simulink model "ElectricalThermalSystemSSC"  (R2026b)
settings: Solver=VariableStepAuto
undefined symbols (not defined in the file): coolant_pipe_D, coolant_valve_D_ratio_max, coolant_valve_D_ratio_min, coolant_valve_displacement, EnvAirTemp, EnvGrvty, PlntThrCabCO2Init, PlntThrCabDucArea, PlntThrCabFanMaxFlw, PlntThrCabHtc, PlntThrCabNPass, PlntThrCabRelHInit, PlntThrCabTempAvg, PlntThrChArea, PlntThrCmpMaxSpd, PlntThrCoolTnkArea, PlntThrCoolTnkVol, PlntThrDoorsArea, PlntThrDoorsK, PlntThrDoorsTk, PlntThrExpDia, PlntThrFanMaxSpd, PlntThrFanMechEff, PlntThrFanVolEff, PlntThrGlassArea, PlntThrGlassK, PlntThrGlassTk, PlntThrHeaterMaxPwr, PlntThrHexNTubes, PlntThrHexTubeDia, PlntThrPipeArea, PlntThrPipeDia, PlntThrPmpMaxSpd, PlntThrPTCLimTemp, PlntThrPTCPwrGain, PlntThrRefrigDia, PlntThrRefrigPinit, PlntThrRoofArea, PlntThrRoofK, PlntThrRoofTk, PlntThrValDisp, PlntThrValDratioMax, PlntThrValDratioMin, PlntThrValRefrDisp, PlntThrValRefrDratio, PlntThrValSplMax, ThrmEM1, ThrmEM2, ThrmEM3, ThrmEM4
libraries: fl_lib x149, nesl_utility x81, SimscapeFluids_lib x35, autolibutils x21
(part 4 of 6)

== system ElectricalThermalSystemSSC/Heater ==
  1 : Inport
  Battery Heater : fl_lib/Thermal/Thermal Elements/Thermal Mass  mass_type=foundation.enum.constant_variable.constant  mass=2 kg  sp_heat=447 J/kg/K  mass_min=1e-6 kg  num_ports=foundation.enum.numPorts2.one  m_specify=off  m_priority=High  m=1 kg  m_nominal_specify=off  m_nominal_value=1  m_nominal_unit=kg  T_specify=on  T_priority=High  T=EnvAirTemp K  T_nominal_specify=off  T_nominal_value=1  T_nominal_unit=K  Q_specify=off  Q_priority=None  Q=0 W  Q_nominal_specify=off  Q_nominal_value=1  Q_nominal_unit=W
  Controlled Heat Flow Rate Source : fl_lib/Thermal/Thermal Sources/Controlled Heat Flow Rate Source
  Convective Heat Transfer : fl_lib/Thermal/Thermal Elements/Convective Heat Transfer  thermal_type=foundation.enum.constant_variable.constant  area=PlntThrHeaterJacArea m^2  heat_tr_coeff=PlntThrHeaterCoeff W/(m^2 * K)  min_heat_tr_coeff=1e-3 W/(K*m^2)  T_specify=off  T_priority=None  T=0 K  T_nominal_specify=off  T_nominal_value=1  T_nominal_unit=K  Q_specify=off  Q_priority=None  Q=0 W  Q_nominal_specify=off  Q_nominal_value=1  Q_nominal_unit=W
  Flow Resistance (TL) : fl_lib/Thermal Liquid/Elements/Flow Resistance (TL)  delta_p_nominal=2e-4 MPa  mdot_nominal=0.15 kg/s  area=PlntThrPipeArea m^2  laminar_fraction=1e-3
  Flow Resistance (TL)1 : fl_lib/Thermal Liquid/Elements/Flow Resistance (TL)  delta_p_nominal=2e-4 MPa  mdot_nominal=0.15 kg/s  area=PlntThrPipeArea m^2  laminar_fraction=1e-3
  Heater Coolant Volume : fl_lib/Thermal Liquid/Elements/Constant Volume Chamber (TL)  volume=PlntThrHeaterJacVol m^3  num_ports=foundation.enum.num_ports.two  area_A=PlntThrPipeArea m^2  area_B=PlntThrPipeArea m^2  area_C=0.01 m^2  area_D=0.01 m^2  p_I_specify=on  p_I_priority=High  p_I=EnvAbsPrs Pa  p_I_nominal_specify=off  p_I_nominal_value=1  p_I_nominal_unit=MPa  T_I_specify=on  T_I_priority=High  T_I=EnvAirTemp K  T_I_nominal_specify=off  T_I_nominal_value=1  T_I_nominal_unit=K  u_I_specify=off  u_I_priority=None  u_I=83.90600000000001 kJ/kg  u_I_nominal_specify=off  u_I_nominal_value=1  u_I_nominal_unit=kJ/kg  rho_I_specify=off  rho_I_priority=None  rho_I=998.21 kg/m^3  rho_I_nominal_specify=off  rho_I_nominal_value=1  rho_I_nominal_unit=kg/m^3
  LPF with IC1 : Subsystem  mask{wc=1, InitCond=0, dataType=off}
      mask prompts: wc "Cutoff frequency, wc [rad/s]"; InitCond "Initial condition, InitCond [same as u]"; dataType "Enforce same input data type"
      mask TypeOptions wc: Cont LPF IC/wc
      mask TypeOptions InitCond: Initial Condition/Value
      mask TypeOptions dataType: Cont LPF IC/dataType
  Max Power [W] : Gain  Gain=PlntThrHeaterMaxPwr
  Signal Specification : SignalSpecification  Unit=W
  Simulink-PS Converter : nesl_utility/Simulink-PS Converter  PhysicalDomain=network_engine_domain  SubClassName=ps_input  LeftPortType=input  RightPortType=output  PseudoPeriodic=off  Frequencies=[]  NoiseDistribution=none  NoiseParameters=[]  Unit=W  AffineConversion=off  FilteringAndDerivatives=provide  SimscapeFilterOrder=1  InputFilterTimeConstant=0.001  UdotUserProvided=0
  Thermal Reference : fl_lib/Thermal/Thermal Elements/Thermal Reference
  B : PMIOPort  Side=Left
  A : PMIOPort  Port=2  Side=Right
  01 : Outport
  wires:
  1/1 -> LPF with IC1/1(u)
  LPF with IC1/1(y) -> Max Power [W]/1
  Max Power [W]/1 -> Signal Specification/1, Simulink-PS Converter/1
  Signal Specification/1 -> 01/1
  connections:
  Battery Heater/LConn1 -- Controlled Heat Flow Rate Source/LConn1 -- Convective Heat Transfer/LConn1
  Convective Heat Transfer/RConn1 -- Heater Coolant Volume/LConn2
  Simulink-PS Converter/RConn1 -- Controlled Heat Flow Rate Source/RConn1
  Flow Resistance (TL)/LConn1 -- A/RConn1
  Flow Resistance (TL)1/RConn1 -- B/RConn1
  Flow Resistance (TL)1/LConn1 -- Heater Coolant Volume/RConn1
  Flow Resistance (TL)/RConn1 -- Heater Coolant Volume/LConn1
  Thermal Reference/LConn1 -- Controlled Heat Flow Rate Source/RConn2

== system ElectricalThermalSystemSSC/Inner Condenser ==
  Inner Condenser : SimscapeFluids_lib/Heat Exchangers/Two-Phase Fluid - Moist Air/Condenser Evaporator (2P-MA)  flow_arrangement=fluids.heat_exchangers.enum.FlowArrangement2PMA.Cross  cross_flow_arrangement=fluids.heat_exchangers.enum.CrossFlowArrangement2PMA.UnmixedUnmixed  R_wall=PlntThrICondThermalR K/kW  wall_thermal_mass=false  mass_wall=1 kg  cp_wall=490 J/(K*kg)  area_A1=PlntThrRefrigArea m^2  area_B1=PlntThrRefrigArea m^2  area_A2=PlntThrCabDucArea m^2  area_B2=PlntThrCabDucArea m^2  tube_num_2P=PlntThrICondNTubes  tube_length_2P=PlntThrICondLen m  tube_cross_section_2P=fluids.heat_exchangers.enum.TubeCrossSection.Rectangular  tube_diameter_2P=0.05 m  tube_width_2P=PlntThrICondWdt m  tube_height_2P=PlntThrICondTubHgt m  tube_inner_diameter_2P=0.05 m  tube_outer_diameter_2P=0.1 m  tube_flow_area_2P=0.002 m^2  tube_wetted_perimeter_2P=0.15 m  tube_heat_perimeter_2P=0.15 m  tube_pressure_loss_spec_2P=fluids.heat_exchangers.enum.TubePressureLossSpec2P.Haaland  tube_loss_coeff_2P=10  tube_local_pressure_loss_spec_2P=fluids.heat_exchangers.enum.LocalLossSpec.AggregateLength  tube_length_add_2P=PlntThrICondTubLEq m  tube_local_loss_coefficient_2P=0.1  tube_roughness_pressure_2P=15e-6 m  tube_Re_lam_pressure_2P=2000  tube_Re_tur_pressure_2P=4000  tube_shape_factor_generic_2P=64  tube_heat_coeff_spec_2P=fluids.heat_exchangers.enum.TubeHeatCoeffSpec2P.GneilinskiCavalliniZecchin  tube_colburn_coeff_liq_2P=[.023, .8, .33]  tube_colburn_coeff_mix_2P=[.05, .8, .33]  tube_colburn_coeff_vap_2P=[.023, .8, .33]  tube_roughness_heat_2P=15e-6 m  tube_Re_lam_heat_2P=2000  tube_Re_tur_heat_2P=4000  tube_Nu_lam_generic_2P=3.66  fouling_factor_2P=0.1 K*m^2/kW  fin_area_2P=PlntThrICondTubAWb m^2  fin_efficiency_2P=0.6  energy_spec_2P=foundation.enum.energy_spec.void_fraction  p_init_2P=PlntThrRefrigPinit Pa  T_init_2P=293.15 K  x_init_2P=0.5  alpha_init_2P=PlntThrRefrigAinit  h_init_2P=1500 kJ/kg  u_init_2P=1500 kJ/kg  flow_geometry_MA=fluids.heat_exchangers.enum.FlowGeometryMA.Generic  tube_num_MA=25  tube_length_MA=1 m  tube_cross_section_MA=fluids.heat_exchangers.enum.TubeCrossSection.Circular  tube_diameter_MA=0.05 m  tube_width_MA=0.05 m  tube_height_MA=0.05 m  tube_inner_diameter_MA=0.05 m  tube_outer_diameter_MA=0.1 m  tube_flow_area_MA=0.002 m^2  tube_wetted_perimeter_MA=0.15 m  tube_heat_perimeter_MA=0.15 m  tube_pressure_loss_spec_MA=fluids.heat_exchangers.enum.TubePressureLossSpec.Haaland  tube_loss_coeff_MA=10  tube_local_pressure_loss_spec_MA=fluids.heat_exchangers.enum.LocalLossSpec.AggregateLength  tube_length_add_MA=0.1 m  tube_local_loss_coefficient_MA=0.1  tube_roughness_pressure_MA=15e-6 m  tube_Re_lam_pressure_MA=2000  tube_Re_tur_pressure_MA=4000  tube_shape_factor_generic_MA=64  tube_heat_coeff_spec_MA=fluids.heat_exchangers.enum.TubeHeatCoeffSpec.Gneilinski  tube_colburn_coeff_MA=[.023, .8, .33]  tube_roughness_heat_MA=15e-6 m  tube_Re_lam_heat_MA=2000  tube_Re_tur_heat_MA=4000  tube_Nu_lam_generic_MA=3.66  bank_arrangement_MA=fluids.heat_exchangers.enum.BankArrangement.Inline  bank_num_rows_MA=5  bank_tubes_per_row_MA=5  bank_width_MA=1 m  bank_tube_diameter_MA=0.05 m  bank_longitudinal_pitch_MA=0.15 m  bank_transverse_pitch_MA=0.15 m  bank_pressure_loss_spec_MA=fluids.heat_exchangers.enum.BankPressureLossSpec.Martin  bank_euler_MA=10  bank_heat_coeff_spec_MA=fluids.heat_exchangers.enum.BankHeatCoeffSpec.Martin  bank_colburn_coeff_MA=[.27, .63, .36]  generic_flow_area_MA=PlntThrICondAreaFlw m^2  generic_heat_area_MA=PlntThrICondAreaPr m^2  generic_volume_MA=PlntThrICondAirVol m^3  generic_loss_coeff_MA=10  generic_colburn_coeff_MA=[.023, .8, .33]  fouling_factor_MA=0.1 K*m^2/kW  fin_area_MA=PlntThrICondAreaFins m^2  fin_efficiency_MA=0.7  p_init_MA=EnvAbsPrs Pa  T_init_MA=EnvAirTemp K  humidity_spec_MA=foundation.enum.HumiditySpec.RelativeHumidity  RH_init_MA=PlntThrCabRelHInit  x_w_init_MA=0.01  y_w_init_MA=0.01  HR_init_MA=0.01  Tw_init_MA=287 K  trace_gas_spec_MA=foundation.enum.trace_gas_spec.mole_fraction  x_g_init_MA=0.001  y_g_init_MA=PlntThrCabCO2Init  r_d_init_MA=0  RH_ws_MA=1  time_constant_cond_MA=1e-3 s  time_constant_evap_MA=1e-3 s  fraction_entrained_MA=1
  PS-Simulink Converter1 : nesl_utility/PS-Simulink Converter  PhysicalDomain=network_engine_domain  SubClassName=ps_output  LeftPortType=input  RightPortType=output  PseudoPeriodic=off  Frequencies=[]  VectorFormat=inherit  Unit=MPa  AffineConversion=off
  "Pressure, Temperature & Internal Energy Sensor (2P)" : fl_lib/Two-Phase Fluid/Sensors/Pressure, Temperature & Internal Energy Sensor (2P)  reference=foundation.enum.MeasurementReference.absolute  pressure=true  pressure_spec=foundation.enum.PressureMeasementSpec.Absolute  temperature=false  internal_energy=false
  C : PMIOPort  Side=Left
  B : PMIOPort  Port=2  Side=Left
  D : PMIOPort  Port=3  Side=Right
  A : PMIOPort  Port=4  Side=Right
  01 : Outport
  wires:
  PS-Simulink Converter1/1 -> 01/1
  connections:
  PS-Simulink Converter1/LConn1 -- "Pressure, Temperature & Internal Energy Sensor (2P)"/RConn1
  Inner Condenser/LConn3 -- B/RConn1 -- "Pressure, Temperature & Internal Energy Sensor (2P)"/LConn1
  A/RConn1 -- Inner Condenser/LConn1
  C/RConn1 -- Inner Condenser/RConn3
  D/RConn1 -- Inner Condenser/RConn1

== system ElectricalThermalSystemSSC/LPF with IC1 ==
  u : Inport
  Cont LPF IC : autolibutils/Cont LPF IC  wc=wc  aMode=1  dataType=off
  Initial Condition : Constant  Value=InitCond  SampleTime=-1
  y : Outport
  wires:
  Initial Condition/1 -> Cont LPF IC/2
  u/1 -> Cont LPF IC/1
  Cont LPF IC/1 -> y/1

== system ElectricalThermalSystemSSC/Motor ==
  Cooling Assembly : Subsystem  Variant=on  VariantControl=Cooling Assembly  EmptyChoice=on
  PS-Simulink Converter : nesl_utility/PS-Simulink Converter  PhysicalDomain=network_engine_domain  SubClassName=ps_output  LeftPortType=input  RightPortType=output  PseudoPeriodic=off  Frequencies=[]  VectorFormat=inherit  Unit=K  AffineConversion=on
  Pressure & Temperature Sensor (TL) : fl_lib/Thermal Liquid/Sensors/Pressure & Temperature Sensor (TL)  reference=foundation.enum.MeasurementReference.absolute  pressure=false  pressure_spec=foundation.enum.PressureMeasementSpec.Absolute  temperature=true
  Simscape Bus1 : SimscapeBus  HierarchyStrings=ThrmEM4;ThrmEM3;ThrmEM2;ThrmEM1
  A : PMIOPort  Side=Left
  B : PMIOPort  Port=2  Side=Right
  T : PMIOPort  Port=3  Side=Right
  01 : Outport
  02 : Outport  Port=2
  03 : Outport  Port=3
  wires:
  Cooling Assembly/2(Qem) -> 03/1
  PS-Simulink Converter/1 -> 02/1
  Cooling Assembly/1(EMTemp) -> 01/1
  connections:
  Simscape Bus1/LConn1 -- Cooling Assembly/RConn2
  Simscape Bus1/LConn4 -- Cooling Assembly/RConn5
  Simscape Bus1/LConn3 -- Cooling Assembly/RConn4
  Pressure & Temperature Sensor (TL)/LConn1 -- B/RConn1 -- Cooling Assembly/RConn1
  T/RConn1 -- Simscape Bus1/RConn1
  A/RConn1 -- Cooling Assembly/LConn1
  Simscape Bus1/LConn2 -- Cooling Assembly/RConn3
  PS-Simulink Converter/LConn1 -- Pressure & Temperature Sensor (TL)/RConn1

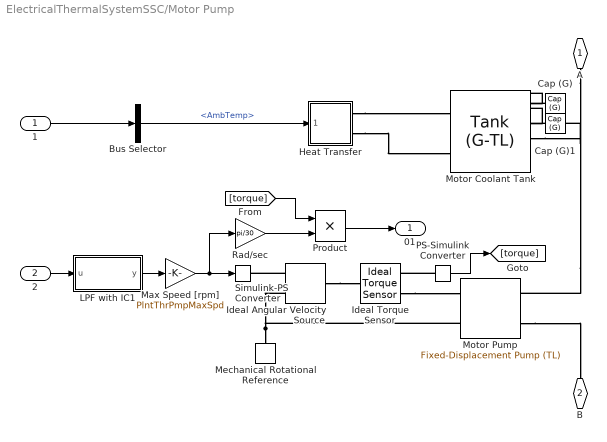
== system ElectricalThermalSystemSSC/Motor Pump ==
  1 : Inport
  2 : Inport  Port=2
  Bus Selector : BusSelector  OutputSignals=AmbTemp
  Cap (G) : fl_lib/Gas/Elements/Cap (G)  p_specify=off  p_priority=None  p=0.101325 MPa  p_nominal_specify=off  p_nominal_value=1  p_nominal_unit=MPa  T_specify=off  T_priority=None  T=293.15 K  T_nominal_specify=off  T_nominal_value=1  T_nominal_unit=K
  Cap (G)1 : fl_lib/Gas/Elements/Cap (G)  p_specify=off  p_priority=None  p=0.101325 MPa  p_nominal_specify=off  p_nominal_value=1  p_nominal_unit=MPa  T_specify=off  T_priority=None  T=293.15 K  T_nominal_specify=off  T_nominal_value=1  T_nominal_unit=K
  Heat Transfer : Subsystem
  Ideal Angular Velocity Source : fl_lib/Mechanical/Mechanical Sources/Ideal Angular Velocity Source
  Ideal Torque Sensor : fl_lib/Mechanical/Mechanical Sensors/Ideal Torque Sensor
  LPF with IC1 : Subsystem  mask{wc=1, InitCond=0, dataType=off}
      mask prompts: wc "Cutoff frequency, wc [rad/s]"; InitCond "Initial condition, InitCond [same as u]"; dataType "Enforce same input data type"
      mask TypeOptions wc: Cont LPF IC/wc
      mask TypeOptions InitCond: Initial Condition/Value
      mask TypeOptions dataType: Cont LPF IC/dataType
  Max Speed [rpm] : Gain  Gain=PlntThrPmpMaxSpd
  Mechanical Rotational Reference : fl_lib/Mechanical/Rotational Elements/Mechanical Rotational Reference
  Motor Coolant Tank : SimscapeFluids_lib/Thermal Liquid/Tanks & Accumulators/Tank (G-TL)  num_inlet=2  volume_total=PlntThrCoolTnkVol l  volume_spec=1  tank_area=PlntThrCoolTnkArea m^2  level_TLU=[0, 3, 5] m  volume_TLU=[0, 4, 6] m^3  inlet_areas_A1B1=[.01, .01] m^2  inlet_height_A2=0.1 m  inlet_area_A2=0.01 m^2  inlet_heights_A2B2=[0, 0] m  inlet_areas_A2B2=[1 1] *PlntThrPipeArea m^2  inlet_heights_A2B2C2=[.1, .05, 0] m  inlet_areas_A2B2C2=[.01, .01, .01] m^2  inlet_heights_A2B2C2D2=0.1 * ones(1, 4) m  inlet_areas_A2B2C2D2=0.01 * ones(1, 4) m^2  inlet_heights_A2B2C2D2E2=0.1 * ones(1, 5) m  inlet_areas_A2B2C2D2E2=0.01 * ones(1, 5) m^2  inlet_heights_A2B2C2D2E2F2=0.1 * ones(1, 6) m  inlet_areas_A2B2C2D2E2F2=0.01 * ones(1, 6) m^2  capacity_check=0  max_liquid_capacity=coolant_tank_volume l  g=0 m/s^2  level_specify=on  level_priority=None  level=5 m  level_nominal_specify=off  level_nominal_value=1  level_nominal_unit=m  volume_liquid_specify=on  volume_liquid_priority=High  volume_liquid=0.5 * PlntThrCoolTnkVol l  volume_liquid_nominal_specify=off  volume_liquid_nominal_value=1  volume_liquid_nominal_unit=m^3  mass_liquid_specify=off  mass_liquid_priority=None  mass_liquid=5e+3 kg  mass_liquid_nominal_specify=off  mass_liquid_nominal_value=1  mass_liquid_nominal_unit=kg  T_liquid_specify=on  T_liquid_priority=High  T_liquid=EnvAirTemp K  T_liquid_nominal_specify=off  T_liquid_nominal_value=1  T_liquid_nominal_unit=K  p_gas_specify=on  p_gas_priority=High  p_gas=EnvAbsPrs Pa  p_gas_nominal_specify=off  p_gas_nominal_value=1  p_gas_nominal_unit=MPa  T_gas_specify=on  T_gas_priority=High  T_gas=EnvAirTemp K  T_gas_nominal_specify=off  T_gas_nominal_value=1  T_gas_nominal_unit=K  rho_gas_specify=off  rho_gas_priority=None  rho_gas=1.2 kg/m^3  rho_gas_nominal_specify=off  rho_gas_nominal_value=1  rho_gas_nominal_unit=kg/m^3
  Motor Pump : SimscapeFluids_lib/Thermal Liquid/Pumps & Motors/Fixed-Displacement Pump (TL)  loss_spec=1  displacement=PlntThrPmpDisp l/rev  omega_nominal=0.5 * PlntThrPmpMaxSpd rpm  p_nominal=0.1 MPa  mu_nominal=0.9 cP  vol_eff_nominal=0.92  mech_eff_nominal=0.88  no_load_torque=0.03 N*m  p_diff_eff_TLU=[.1, 1, 2] MPa  omega_eff_TLU=[25, 50, 100, 200, 300, 400] rad/s  vol_eff_TLU=[.816, .908, .954, .977, .981, .984; .325, .663, .831, .916, .925, .946; .137, .568, .78, .892, .893, .91]  mech_eff_TLU=[.996, .996, .996, .996, .996, .996; .988, .989, .989, .989, .989, .99; .981, .981, .982, .982, .983, .984]  p_diff_loss_TLU=[.1, 1, 2] MPa  omega_loss_TLU=[25, 50, 100, 200, 300, 400] rad/s  vol_loss_TLU=[.023, .023, .023, .023, .0285, .032; .0844, .0842, .0845, .084, .1125, .108; .1079, .108, .11, .108, .1605, .18] * 1e-3 m^3/s  mech_loss_TLU=[.002, .002, .002, .002, .002, .002; .0607, .0556, .0556, .0556, .0556, .0505; .1937, .1937, .1833, .1833, .1729, .1626] N*m  vol_eff_min=1e-3  vol_eff_max=1  mech_eff_min=1e-3  mech_eff_max=1  pressure_threshold=1e-3 MPa  omega_threshold=10 rad/s  area=PlntThrPipeArea m^2  supplied_range_check=0  pump_mode_check=simscape.enum.assert.action.none  pressure_check=simscape.enum.assert.action.none  p_min_valid=0.101325 MPa
  PS-Simulink Converter : nesl_utility/PS-Simulink Converter  PhysicalDomain=network_engine_domain  SubClassName=ps_output  LeftPortType=input  RightPortType=output  PseudoPeriodic=off  Frequencies=[]  VectorFormat=inherit  Unit=N*m  AffineConversion=off
  Product : Product
  Rad/sec : Gain  Gain=pi/30
  Simulink-PS Converter : nesl_utility/Simulink-PS Converter  PhysicalDomain=network_engine_domain  SubClassName=ps_input  LeftPortType=input  RightPortType=output  PseudoPeriodic=off  Frequencies=[]  NoiseDistribution=none  NoiseParameters=[]  Unit=rpm  AffineConversion=off  FilteringAndDerivatives=provide  SimscapeFilterOrder=1  InputFilterTimeConstant=0.001  UdotUserProvided=0
  A : PMIOPort  Side=Left
  B : PMIOPort  Port=2  Side=Right
  01 : Outport
  wires:
  2/1 -> LPF with IC1/1(u)
  Bus Selector/1 -> Heat Transfer/1(1)  "<AmbTemp>"
  1/1 -> Bus Selector/1
  LPF with IC1/1(y) -> Max Speed [rpm]/1
  Max Speed [rpm]/1 -> Rad/sec/1, Simulink-PS Converter/1
  PS-Simulink Converter/1 -> [torque]
  Rad/sec/1 -> Product/2
  [torque] -> Product/1
  Product/1 -> 01/1
  connections:
  Mechanical Rotational Reference/LConn1 -- Ideal Angular Velocity Source/RConn2 -- Motor Pump/RConn2
  Motor Pump/LConn2 -- B/RConn1
  Heat Transfer/RConn2 -- Motor Coolant Tank/RConn2
  Cap (G)/LConn1 -- Motor Coolant Tank/LConn1
  Heat Transfer/RConn1 -- Motor Coolant Tank/RConn1
  Motor Coolant Tank/LConn4 -- Motor Pump/LConn1
  A/RConn1 -- Motor Coolant Tank/LConn3
  Cap (G)1/LConn1 -- Motor Coolant Tank/LConn2
  Ideal Angular Velocity Source/RConn1 -- Simulink-PS Converter/RConn1
  Ideal Torque Sensor/RConn1 -- Motor Pump/RConn1
  Ideal Angular Velocity Source/LConn1 -- Ideal Torque Sensor/LConn1
  PS-Simulink Converter/LConn1 -- Ideal Torque Sensor/RConn2

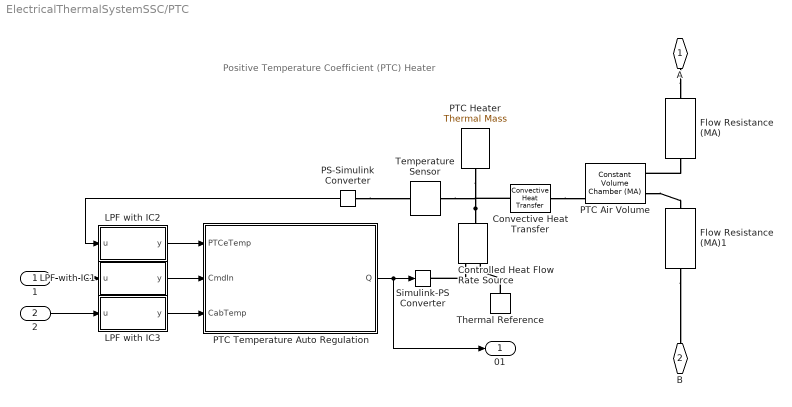
== system ElectricalThermalSystemSSC/PTC ==
  note: Positive Temperature Coefficient (PTC) Heater
  1 : Inport
  2 : Inport  Port=2
  Controlled Heat Flow Rate Source : fl_lib/Thermal/Thermal Sources/Controlled Heat Flow Rate Source
  Convective Heat Transfer : fl_lib/Thermal/Thermal Elements/Convective Heat Transfer  thermal_type=foundation.enum.constant_variable.constant  area=PlntThrPTCArea m^2  heat_tr_coeff=PlntThrPTCHtc W/(m^2 * K)  min_heat_tr_coeff=1e-3 W/(K*m^2)  T_specify=off  T_priority=None  T=0 K  T_nominal_specify=off  T_nominal_value=1  T_nominal_unit=K  Q_specify=off  Q_priority=None  Q=0 W  Q_nominal_specify=off  Q_nominal_value=1  Q_nominal_unit=W
  Flow Resistance (MA) : fl_lib/Moist Air/Elements/Flow Resistance (MA)  delta_p_nominal=2e-4 MPa  mdot_nominal=0.15 kg/s  rho_nominal=1.2 kg/m^3  area=PlntThrCabDucArea m^2  laminar_fraction=1e-3
  Flow Resistance (MA)1 : fl_lib/Moist Air/Elements/Flow Resistance (MA)  delta_p_nominal=2e-4 MPa  mdot_nominal=0.15 kg/s  rho_nominal=1.2 kg/m^3  area=PlntThrCabDucArea m^2  laminar_fraction=1e-3
  LPF with IC1 : Subsystem  mask{wc=1, InitCond=0, dataType=off}
      mask prompts: wc "Cutoff frequency, wc [rad/s]"; InitCond "Initial condition, InitCond [same as u]"; dataType "Enforce same input data type"
      mask TypeOptions wc: Cont LPF IC/wc
      mask TypeOptions InitCond: Initial Condition/Value
      mask TypeOptions dataType: Cont LPF IC/dataType
  LPF with IC2 : Subsystem  mask{wc=10, InitCond=0, dataType=off}
      mask prompts: wc "Cutoff frequency, wc [rad/s]"; InitCond "Initial condition, InitCond [same as u]"; dataType "Enforce same input data type"
      mask TypeOptions wc: Cont LPF IC/wc
      mask TypeOptions InitCond: Initial Condition/Value
      mask TypeOptions dataType: Cont LPF IC/dataType
  LPF with IC3 : Subsystem  mask{wc=1, InitCond=0, dataType=off}
      mask prompts: wc "Cutoff frequency, wc [rad/s]"; InitCond "Initial condition, InitCond [same as u]"; dataType "Enforce same input data type"
      mask TypeOptions wc: Cont LPF IC/wc
      mask TypeOptions InitCond: Initial Condition/Value
      mask TypeOptions dataType: Cont LPF IC/dataType
  PS-Simulink Converter : nesl_utility/PS-Simulink Converter  PhysicalDomain=network_engine_domain  SubClassName=ps_output  LeftPortType=input  RightPortType=output  PseudoPeriodic=off  Frequencies=[]  VectorFormat=inherit  Unit=inherit  AffineConversion=off
  PTC Heater : fl_lib/Thermal/Thermal Elements/Thermal Mass  mass_type=foundation.enum.constant_variable.constant  mass=PlntThrPTCmass kg  sp_heat=PlntThrPTCCp J/kg/K  mass_min=1e-6 kg  num_ports=foundation.enum.numPorts2.one  m_specify=off  m_priority=High  m=1 kg  m_nominal_specify=off  m_nominal_value=1  m_nominal_unit=kg  T_specify=on  T_priority=High  T=EnvAirTemp K  T_nominal_specify=off  T_nominal_value=1  T_nominal_unit=K  Q_specify=off  Q_priority=None  Q=0 W  Q_nominal_specify=off  Q_nominal_value=1  Q_nominal_unit=W
  PTC Air Volume : fl_lib/Moist Air/Elements/Constant Volume Chamber (MA)  volume=0.001 m^3  num_ports=foundation.enum.num_ports.two  area_A=PlntThrCabDucArea m^2  area_B=PlntThrCabDucArea m^2  area_C=0.01 m^2  area_D=0.01 m^2  RH_ws=1  time_constant_cond=1e-3 s  time_constant_evap=1e-3 s  fraction_entrained=1  moisture_trace_gas_source=foundation.enum.moisture_trace_gas_source.none  moisture_source_spec=foundation.enum.MoistureSourceSpec.WaterVapor  vapor_from_liquid=false  moisture_mass_flow=0 kg/s  moisture_temperature_spec=foundation.enum.temperature_spec.atmospheric  moisture_temperature=293.15 K  trace_gas_mass_flow=0 kg/s  trace_gas_temperature_spec=foundation.enum.temperature_spec.atmospheric  trace_gas_temperature=293.15 K  p_init=EnvAbsPrs Pa  p_init_priority=foundation.enum.Priority.High  T_init=EnvAirTemp K  T_init_priority=foundation.enum.Priority.High  humidity_spec=foundation.enum.HumiditySpec.RelativeHumidity  RH_init=PlntThrCabRelHInit  RH_init_priority=foundation.enum.Priority.High  x_w_init=0  x_w_init_priority=foundation.enum.Priority.None  y_w_init=0  y_w_init_priority=foundation.enum.Priority.None  HR_init=0  HR_init_priority=foundation.enum.Priority.None  Tw_init=287 K  Tw_init_priority=foundation.enum.Priority.High  trace_gas_spec=foundation.enum.trace_gas_spec.mole_fraction  x_g_init=0  x_g_init_priority=foundation.enum.Priority.None  y_g_init=PlntThrCabCO2Init  y_g_init_priority=foundation.enum.Priority.High  r_d_init=0  r_d_init_priority=foundation.enum.Priority.High
  PTC Temperature Auto Regulation : Subsystem
  Simulink-PS Converter : nesl_utility/Simulink-PS Converter  PhysicalDomain=network_engine_domain  SubClassName=ps_input  LeftPortType=input  RightPortType=output  PseudoPeriodic=off  Frequencies=[]  NoiseDistribution=none  NoiseParameters=[]  Unit=1  AffineConversion=off  FilteringAndDerivatives=provide  SimscapeFilterOrder=1  InputFilterTimeConstant=0.001  UdotUserProvided=0
  Temperature Sensor : fl_lib/Thermal/Thermal Sensors/Temperature Sensor  temperature_measure=foundation.enum.MeasurementReference.absolute
  Thermal Reference : fl_lib/Thermal/Thermal Elements/Thermal Reference
  A : PMIOPort  Side=Left
  B : PMIOPort  Port=2  Side=Right
  01 : Outport
  wires:
  PTC Temperature Auto Regulation/1(Q) -> 01/1, Simulink-PS Converter/1
  PS-Simulink Converter/1 -> LPF with IC2/1(u)
  1/1 -> LPF with IC1/1(u)
  LPF with IC1/1(y) -> PTC Temperature Auto Regulation/2(CmdIn)
  LPF with IC2/1(y) -> PTC Temperature Auto Regulation/1(PTCeTemp)
  2/1 -> LPF with IC3/1(u)
  LPF with IC3/1(y) -> PTC Temperature Auto Regulation/3(CabTemp)
  connections:
  Controlled Heat Flow Rate Source/RConn1 -- Simulink-PS Converter/RConn1
  PS-Simulink Converter/LConn1 -- Temperature Sensor/RConn1
  A/RConn1 -- Flow Resistance (MA)/LConn1
  PTC Air Volume/LConn2 -- Flow Resistance (MA)1/LConn1
  Flow Resistance (MA)/RConn1 -- PTC Air Volume/LConn1
  Convective Heat Transfer/RConn1 -- PTC Air Volume/RConn3
  Flow Resistance (MA)1/RConn1 -- B/RConn1
  Thermal Reference/LConn1 -- Controlled Heat Flow Rate Source/RConn2
  Controlled Heat Flow Rate Source/LConn1 -- Convective Heat Transfer/LConn1 -- PTC Heater/LConn1 -- Temperature Sensor/LConn1

== system ElectricalThermalSystemSSC/Parallel-Serial Mode Valve 1 ==
  note: Parallel mode flow path: A-C
      | Serial mode flow path: A-B
  1 : Inport
  Bias : Bias  Bias=-1  SaturateOnIntegerOverflow=off
  Gain : Gain  Gain=2
  LPF with IC1 : Subsystem  mask{wc=1, InitCond=0, dataType=off}
      mask prompts: wc "Cutoff frequency, wc [rad/s]"; InitCond "Initial condition, InitCond [same as u]"; dataType "Enforce same input data type"
      mask TypeOptions wc: Cont LPF IC/wc
      mask TypeOptions InitCond: Initial Condition/Value
      mask TypeOptions dataType: Cont LPF IC/dataType
  Max Valve Displacement [m] : Gain  Gain=PlntThrValDisp
  Parallel-Serial Mode Valve : SimscapeFluids_lib/Thermal Liquid/Valves & Orifices/Directional Control Valves/3-Way Directional Valve (TL)  open_orifices_pos=fluids.thermal_liquid.valves.directional_control_valves.enum.OpenOrifices3Way.PA  open_orifices_neg=fluids.thermal_liquid.valves.directional_control_valves.enum.OpenOrifices3Way.AT  area_spec=fluids.thermal_liquid.valves.directional_control_valves.enum.area_spec.identical  valve_spec=fluids.thermal_liquid.valves.enum.orifice_spec.linear  del_S_max=PlntThrValDisp m  area_max=pi * (PlntThrValDratioMax*PlntThrPipeDia)^2 / 4 m^2  del_S_TLU=[0 0.002 0.004 0.007 0.017] m  valve_area_TLU=[1e-09, 2.0352e-07, 4.0736e-05, .00011438, .00034356] m^2  del_S_flow_TLU=[0 0.002 0.004 0.007 0.017] m  p_diff_TLU=[-.1, .3, .5, .7] MPa  vol_flow_TLU=1e-3 * [1.7e-05, 2e-05, 2.6e-05; .0035, .0045, .0053; .7, .9, 1.06; 1.96, 2.5, 3; 6, 7.7, 9.13] m^3/s  mdot_TLU=[-1e-05, 1.7e-05, 2e-05, 2.6e-05; -.002, .0035, .0045, .0053; -.4, .7, .9, 1.06; -1.13, 1.96, 2.5, 3; -3.45, 6, 7.7, 9.13] kg/s  T_ref_in=293.15 K  p_ref_in=0.101325 MPa  area_leak=pi * (PlntThrValDratioMin*PlntThrPipeDia)^2 / 4 m^2  Cd=0.7  Re_c=150  smoothing_factor=0.01  pressure_recovery=simscape.enum.onoff.on  area=PlntThrPipeArea m^2  S_max_PA=PlntThrValSplMax m  del_S_max_PA=coolant_valve_displacement-(coolant_valve_displacement)*(pi * (coolant_valve_D_ratio_min*coolant_pipe_D)^2 / 4)/(pi * (coolant_valve_D_ratio_max*coolant_pipe_D)^2 / 4) m  area_max_PA=pi * (coolant_valve_D_ratio_max*coolant_pipe_D)^2 / 4 m^2  del_S_TLU_PA=[0 0.002 0.004 0.007 0.017] m  valve_area_TLU_PA=[1e-09, 2.0352e-07, 4.0736e-05, .00011438, .00034356] m^2  del_S_flow_TLU_PA=[0 0.002 0.004 0.007 0.017] m  p_diff_TLU_PA=[-.1, .3, .5, .7] MPa  vol_flow_TLU_PA=1e-3 * [1.7e-05, 2e-05, 2.6e-05; .0035, .0045, .0053; .7, .9, 1.06; 1.96, 2.5, 3; 6, 7.7, 9.13] m^3/s  mdot_TLU_PA=[-1e-05, 1.7e-05, 2e-05, 2.6e-05; -.002, .0035, .0045, .0053; -.4, .7, .9, 1.06; -1.13, 1.96, 2.5, 3; -3.45, 6, 7.7, 9.13] kg/s  S_max_AT=-PlntThrValSplMax m  del_S_max_AT=coolant_valve_displacement-(coolant_valve_displacement)*(pi * (coolant_valve_D_ratio_min*coolant_pipe_D)^2 / 4)/(pi * (coolant_valve_D_ratio_max*coolant_pipe_D)^2 / 4) m  area_max_AT=pi * (coolant_valve_D_ratio_max*coolant_pipe_D)^2 / 4 m^2  del_S_TLU_AT=[0 0.002 0.004 0.007 0.017] m  valve_area_TLU_AT=[1e-09, 2.0352e-07, 4.0736e-05, .00011438, .00034356] m^2  del_S_flow_TLU_AT=[0 0.002 0.004 0.007 0.017] m  p_diff_TLU_AT=[-.1, .3, .5, .7] MPa  vol_flow_TLU_AT=1e-3 * [1.7e-05, 2e-05, 2.6e-05; .0035, .0045, .0053; .7, .9, 1.06; 1.96, 2.5, 3; 6, 7.7, 9.13] m^3/s  mdot_TLU_AT=[-1e-05, 1.7e-05, 2e-05, 2.6e-05; -.002, .0035, .0045, .0053; -.4, .7, .9, 1.06; -1.13, 1.96, 2.5, 3; -3.45, 6, 7.7, 9.13] kg/s  S_max_PT=2.5e-3 m  del_S_max_PT=0.005 m  area_max_PT=1e-4 m^2  del_S_TLU_PT=[0, .002, .004, .007, .017] m  valve_area_TLU_PT=[1e-09, 2.0352e-07, 4.0736e-05, .00011438, .00034356] m^2  del_S_flow_TLU_PT=[0, .002, .004, .007, .017] m  p_diff_TLU_PT=[.3, .5, .7] MPa  vol_flow_TLU_PT=1e-3 * [1.7e-05, 2e-05, 2.6e-05; .0035, .0045, .0053; .7, .9, 1.06; 1.96, 2.5, 3; 6, 7.7, 9.13] m^3/s  mdot_TLU_PT=[1.7e-05, 2e-05, 2.6e-05; .0035, .0045, .0053; .7, .9, 1.06; 1.96, 2.5, 3; 6, 7.7, 9.13] kg/s
  Simulink-PS Converter : nesl_utility/Simulink-PS Converter  PhysicalDomain=network_engine_domain  SubClassName=ps_input  LeftPortType=input  RightPortType=output  PseudoPeriodic=off  Frequencies=[]  NoiseDistribution=none  NoiseParameters=[]  Unit=m  AffineConversion=off  FilteringAndDerivatives=provide  SimscapeFilterOrder=1  InputFilterTimeConstant=0.001  UdotUserProvided=0
  C : PMIOPort  Side=Left
  A : PMIOPort  Port=2  Side=Right
  B : PMIOPort  Port=3  Side=Right
  wires:
  1/1 -> LPF with IC1/1(u)
  Gain/1 -> Bias/1
  LPF with IC1/1(y) -> Gain/1
  Max Valve Displacement [m]/1 -> Simulink-PS Converter/1
  Bias/1 -> Max Valve Displacement [m]/1
  connections:
  Parallel-Serial Mode Valve/RConn1 -- Simulink-PS Converter/RConn1
  Parallel-Serial Mode Valve/RConn3 -- C/RConn1
  Parallel-Serial Mode Valve/LConn1 -- A/RConn1
  Parallel-Serial Mode Valve/RConn2 -- B/RConn1

== system ElectricalThermalSystemSSC/Parallel-Serial Mode Valve 2 ==
  note: Parallel mode flow path: A-C
      | Serial mode flow path: A-B
  1 : Inport
  Bias : Bias  Bias=-1  SaturateOnIntegerOverflow=off
  Gain : Gain  Gain=2
  LPF with IC1 : Subsystem  mask{wc=1, InitCond=0, dataType=off}
      mask prompts: wc "Cutoff frequency, wc [rad/s]"; InitCond "Initial condition, InitCond [same as u]"; dataType "Enforce same input data type"
      mask TypeOptions wc: Cont LPF IC/wc
      mask TypeOptions InitCond: Initial Condition/Value
      mask TypeOptions dataType: Cont LPF IC/dataType
  Max Valve Displacement [m] : Gain  Gain=PlntThrValDisp
  Parallel-Serial Mode Valve : SimscapeFluids_lib/Thermal Liquid/Valves & Orifices/Directional Control Valves/3-Way Directional Valve (TL)  open_orifices_pos=fluids.thermal_liquid.valves.directional_control_valves.enum.OpenOrifices3Way.PA  open_orifices_neg=fluids.thermal_liquid.valves.directional_control_valves.enum.OpenOrifices3Way.AT  area_spec=fluids.thermal_liquid.valves.directional_control_valves.enum.area_spec.identical  valve_spec=fluids.thermal_liquid.valves.enum.orifice_spec.linear  del_S_max=PlntThrValDisp m  area_max=pi * (PlntThrValDratioMax*PlntThrPipeDia)^2 / 4 m^2  del_S_TLU=[0 0.002 0.004 0.007 0.017] m  valve_area_TLU=[1e-09, 2.0352e-07, 4.0736e-05, .00011438, .00034356] m^2  del_S_flow_TLU=[0 0.002 0.004 0.007 0.017] m  p_diff_TLU=[-.1, .3, .5, .7] MPa  vol_flow_TLU=1e-3 * [1.7e-05, 2e-05, 2.6e-05; .0035, .0045, .0053; .7, .9, 1.06; 1.96, 2.5, 3; 6, 7.7, 9.13] m^3/s  mdot_TLU=[-1e-05, 1.7e-05, 2e-05, 2.6e-05; -.002, .0035, .0045, .0053; -.4, .7, .9, 1.06; -1.13, 1.96, 2.5, 3; -3.45, 6, 7.7, 9.13] kg/s  T_ref_in=293.15 K  p_ref_in=0.101325 MPa  area_leak=pi * (PlntThrValDratioMin*PlntThrPipeDia)^2 / 4 m^2  Cd=0.7  Re_c=150  smoothing_factor=0.01  pressure_recovery=simscape.enum.onoff.on  area=PlntThrPipeArea m^2  S_max_PA=PlntThrValSplMax m  del_S_max_PA=coolant_valve_displacement-(coolant_valve_displacement)*(pi * (coolant_valve_D_ratio_min*coolant_pipe_D)^2 / 4)/(pi * (coolant_valve_D_ratio_max*coolant_pipe_D)^2 / 4) m  area_max_PA=pi * (coolant_valve_D_ratio_max*coolant_pipe_D)^2 / 4 m^2  del_S_TLU_PA=[0 0.002 0.004 0.007 0.017] m  valve_area_TLU_PA=[1e-09, 2.0352e-07, 4.0736e-05, .00011438, .00034356] m^2  del_S_flow_TLU_PA=[0 0.002 0.004 0.007 0.017] m  p_diff_TLU_PA=[-.1, .3, .5, .7] MPa  vol_flow_TLU_PA=1e-3 * [1.7e-05, 2e-05, 2.6e-05; .0035, .0045, .0053; .7, .9, 1.06; 1.96, 2.5, 3; 6, 7.7, 9.13] m^3/s  mdot_TLU_PA=[-1e-05, 1.7e-05, 2e-05, 2.6e-05; -.002, .0035, .0045, .0053; -.4, .7, .9, 1.06; -1.13, 1.96, 2.5, 3; -3.45, 6, 7.7, 9.13] kg/s  S_max_AT=-PlntThrValSplMax m  del_S_max_AT=coolant_valve_displacement-(coolant_valve_displacement)*(pi * (coolant_valve_D_ratio_min*coolant_pipe_D)^2 / 4)/(pi * (coolant_valve_D_ratio_max*coolant_pipe_D)^2 / 4) m  area_max_AT=pi * (coolant_valve_D_ratio_max*coolant_pipe_D)^2 / 4 m^2  del_S_TLU_AT=[0 0.002 0.004 0.007 0.017] m  valve_area_TLU_AT=[1e-09, 2.0352e-07, 4.0736e-05, .00011438, .00034356] m^2  del_S_flow_TLU_AT=[0 0.002 0.004 0.007 0.017] m  p_diff_TLU_AT=[-.1, .3, .5, .7] MPa  vol_flow_TLU_AT=1e-3 * [1.7e-05, 2e-05, 2.6e-05; .0035, .0045, .0053; .7, .9, 1.06; 1.96, 2.5, 3; 6, 7.7, 9.13] m^3/s  mdot_TLU_AT=[-1e-05, 1.7e-05, 2e-05, 2.6e-05; -.002, .0035, .0045, .0053; -.4, .7, .9, 1.06; -1.13, 1.96, 2.5, 3; -3.45, 6, 7.7, 9.13] kg/s  S_max_PT=2.5e-3 m  del_S_max_PT=0.005 m  area_max_PT=1e-4 m^2  del_S_TLU_PT=[0, .002, .004, .007, .017] m  valve_area_TLU_PT=[1e-09, 2.0352e-07, 4.0736e-05, .00011438, .00034356] m^2  del_S_flow_TLU_PT=[0, .002, .004, .007, .017] m  p_diff_TLU_PT=[.3, .5, .7] MPa  vol_flow_TLU_PT=1e-3 * [1.7e-05, 2e-05, 2.6e-05; .0035, .0045, .0053; .7, .9, 1.06; 1.96, 2.5, 3; 6, 7.7, 9.13] m^3/s  mdot_TLU_PT=[1.7e-05, 2e-05, 2.6e-05; .0035, .0045, .0053; .7, .9, 1.06; 1.96, 2.5, 3; 6, 7.7, 9.13] kg/s
  Simulink-PS Converter : nesl_utility/Simulink-PS Converter  PhysicalDomain=network_engine_domain  SubClassName=ps_input  LeftPortType=input  RightPortType=output  PseudoPeriodic=off  Frequencies=[]  NoiseDistribution=none  NoiseParameters=[]  Unit=m  AffineConversion=off  FilteringAndDerivatives=provide  SimscapeFilterOrder=1  InputFilterTimeConstant=0.001  UdotUserProvided=0
  A : PMIOPort  Side=Left
  B : PMIOPort  Port=2  Side=Left
  C : PMIOPort  Port=3  Side=Right
  wires:
  1/1 -> LPF with IC1/1(u)
  Bias/1 -> Max Valve Displacement [m]/1
  Gain/1 -> Bias/1
  Max Valve Displacement [m]/1 -> Simulink-PS Converter/1
  LPF with IC1/1(y) -> Gain/1
  connections:
  Parallel-Serial Mode Valve/RConn3 -- C/RConn1
  Parallel-Serial Mode Valve/LConn1 -- A/RConn1
  Parallel-Serial Mode Valve/RConn2 -- B/RConn1
  Simulink-PS Converter/RConn1 -- Parallel-Serial Mode Valve/RConn1

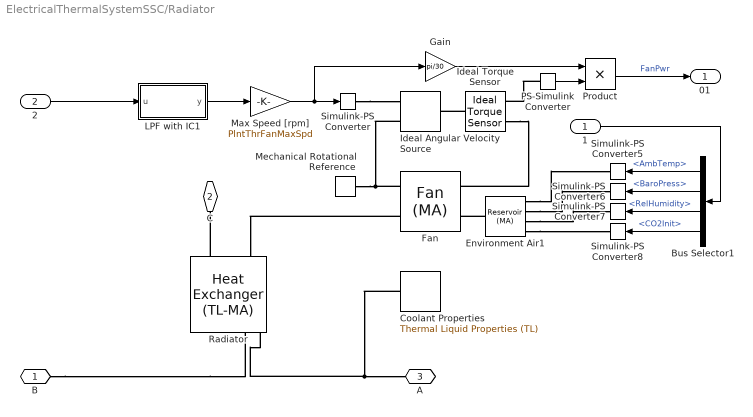
== system ElectricalThermalSystemSSC/Radiator ==
  1 : Inport
  2 : Inport  Port=2
  Bus Selector1 : BusSelector  OutputSignals=AmbTemp,BaroPress,RelHumidity,CO2Init
  Coolant Properties : SimscapeFluids_lib/Thermal Liquid/Utilities/Thermal Liquid Properties (TL)  fluid_list=fluids.thermal_liquid.utilities.enum.thermal_liquid_fluid_list.ethylene_glycol  concentration_param_EG=fluids.thermal_liquid.utilities.enum.thermal_liquid_concentration.volume_fraction  concentration_param_PG=fluids.thermal_liquid.utilities.enum.thermal_liquid_concentration.volume_fraction  c_mass_SW=3.5e-3  c_mass_EG=0.1  c_mass_PG=0.1  c_mass_GL=0.1  c_vol_EG=0.5  c_vol_PG=0.1  beta_const_EG=2.1791 GPa  beta_const_PG=2.1791 GPa  beta_const_GL=2.1791 GPa  p_min_EG=0.01 MPa  p_min_PG=0.01 MPa  p_min_GL=0.01 MPa  p_max_EG=50 MPa  p_max_PG=50 MPa  p_max_GL=50 MPa  T_atm=293.15 K  p_atm=0.101325 MPa  properties_range_check=simscape.enum.assert.action.error  air_fraction=0  R_air=0.287 kJ/(K*kg)  air_dissolution_model=false  p_crit=3 MPa
  Environment Air1 : fl_lib/Moist Air/Elements/Reservoir (MA)  reservoir_spec=foundation.enum.ReservoirSpec.StaticPressureTemperature  pressure_input=true  pressure_spec=foundation.enum.pressure_spec.atmospheric  reservoir_pressure=0.101325 MPa  temperature_input=true  temperature_spec=foundation.enum.temperature_spec.atmospheric  reservoir_temperature=293.15 K  humidity_input=true  humidity_spec=foundation.enum.HumiditySpec.RelativeHumidity  reservoir_RH=0.5  reservoir_x_w=0.01  reservoir_y_w=0.01  reservoir_HR=0.01  reservoir_Tw=287 K  trace_gas_input=true  trace_gas_spec=foundation.enum.trace_gas_spec.mole_fraction  reservoir_x_g=0.001  reservoir_y_g=0.001  water_droplets_input=false  reservoir_r_d=0  RH_ws=1  area_A=PlntThrRadFanAreaFlw m^2  input_error_spec=foundation.enum.input_range_error.warn
  Fan : SimscapeFluids_lib/Moist Air/Turbomachinery/Fan (MA)  fan_parameterization=fluids.moist_air.turbomachinery.enum.FanParameterization.Nominal  mechanical_power_spec=fluids.moist_air.turbomachinery.enum.FanMechanicalPowerSpec.Efficiency  flow_rate_nominal=0.8 m^3/s  pressure_nominal=PlntThrFanNomP Pa  eta_nominal=PlntThrFanVolEff*PlntThrFanMechEff  power_nominal=1620 W  pressure_max=600 Pa  flow_rate_max=1.5 m^3/s  omega_ref_nominal=1000 rpm  flow_rate_1D_TLU=[.0278, .0556, .0833, .111, .139, .167] m^3/s  pressure_1D_TLU=[6410, 6375, 6018, 5366, 4501, 3609] Pa  eta_1D_TLU=[.257, .394, .453, .47, .459, .415]  power_1D_TLU=[693, 900, 1107, 1267, 1363, 1452] W  omega_ref_1D=3000 rpm  rho_ref_1D=1.2 kg/m^3  omega_threshold_factor=1e-2  omega_dp_TLU=[2400; 3000; 3600] rpm  flow_rate_dp_TLU=[.0278, .0556, .0833, .111, .139, .167] m^3/s  pressure_dp_TLU=[4111, 4010, 3551, 2881, 2167, 1453; 6410, 6375, 6018, 5366, 4501, 3609; 9217, 9285, 9022, 8428, 7552, 6482] Pa  eta_dp_TLU=[.3, .434, .468, .459, .4, .3; .257, .394, .453, .47, .459, .415; .225, .359, .434, .461, .47, .459]  power_dp_TLU=[381, 514, 632, 697, 753, 809; 693, 900, 1107, 1267, 1363, 1452; 1139, 1438, 1732, 2029, 2233, 2358] W  rho_ref_dp=1.2 kg/m^3  omega_q_TLU=[2990; 3450; 3867] rpm  pressure_q_TLU=[31, 62, 93, 124] Pa  flow_rate_q_TLU=[.802, .759, .703, .611; .936, .902, .862, .81; 1.056, 1.027, .994, .956] m^3/s  eta_q_TLU=[.088, .162, .22, .261; .068, .128, .18, .222; .055, .105, .148, .188]  power_q_TLU=[283, 290, 297, 290; 427, 437, 445, 452; 595, 606, 625, 631] W  rho_ref_q=1.2 kg/m^3  diameter_ratio=1  mech_orientation=fluids.moist_air.turbomachinery.enum.FanMechanicalOrientation.Positive  area_A=PlntThrRadFanAreaFlw m^2  area_B=PlntThrRadFanAreaFlw m^2
  Gain : Gain  Gain=pi/30
  Ideal Angular Velocity Source : fl_lib/Mechanical/Mechanical Sources/Ideal Angular Velocity Source
  Ideal Torque Sensor : fl_lib/Mechanical/Mechanical Sensors/Ideal Torque Sensor
  LPF with IC1 : Subsystem  mask{wc=1, InitCond=0, dataType=off}
      mask prompts: wc "Cutoff frequency, wc [rad/s]"; InitCond "Initial condition, InitCond [same as u]"; dataType "Enforce same input data type"
      mask TypeOptions wc: Cont LPF IC/wc
      mask TypeOptions InitCond: Initial Condition/Value
      mask TypeOptions dataType: Cont LPF IC/dataType
  Max Speed [rpm] : Gain  Gain=PlntThrFanMaxSpd
  Mechanical Rotational Reference : fl_lib/Mechanical/Rotational Elements/Mechanical Rotational Reference
  PS-Simulink Converter : nesl_utility/PS-Simulink Converter  PhysicalDomain=network_engine_domain  SubClassName=ps_output  LeftPortType=input  RightPortType=output  PseudoPeriodic=off  Frequencies=[]  VectorFormat=inherit  Unit=N*m  AffineConversion=off
  Product : Product
  Radiator : SimscapeFluids_lib/Heat Exchangers/Thermal Liquid - Moist Air/Heat Exchanger (TL-MA)  flow_arrangement=fluids.heat_exchangers.enum.FlowArrangementTLMA.Cross  cross_flow_arrangement=fluids.heat_exchangers.enum.CrossFlowArrangementTLMA.MixedUnmixed  R_wall=PlntThrRadThermalR K/W  wall_thermal_mass=false  mass_wall=1 kg  cp_wall=490 J/(K*kg)  area_A1=PlntThrPipeArea m^2  area_B1=PlntThrPipeArea m^2  area_A2=PlntThrRadAirAreaFlw m^2  area_B2=PlntThrRadAirAreaFlw m^2  flow_geometry_TL=fluids.heat_exchangers.enum.FlowGeometryTL.InsideTubes  tube_num_TL=PlntThrRadNTubes  tube_length_TL=PlntThrRadLength m  tube_cross_section_TL=fluids.heat_exchangers.enum.TubeCrossSection.Rectangular  tube_diameter_TL=0.1 m  tube_width_TL=PlntThrRadWidth m  tube_height_TL=PlntThrRadTubeHeight m  tube_inner_diameter_TL=0.05 m  tube_outer_diameter_TL=0.1 m  tube_flow_area_TL=0.01 m^2  tube_wetted_perimeter_TL=0.4 m  tube_heat_perimeter_TL=0.4 m  tube_pressure_loss_spec_TL=fluids.heat_exchangers.enum.TubePressureLossSpec.Haaland  tube_loss_coeff_TL=10  tube_local_pressure_loss_spec_TL=fluids.heat_exchangers.enum.LocalLossSpec.AggregateLength  tube_length_add_TL=PlntThrRadTubeLEq m  tube_local_loss_coefficient_TL=0.1  tube_roughness_pressure_TL=15e-6 m  tube_Re_lam_pressure_TL=2000  tube_Re_tur_pressure_TL=4000  tube_shape_factor_generic_TL=64  tube_heat_coeff_spec_TL=fluids.heat_exchangers.enum.TubeHeatCoeffSpec.Gneilinski  tube_colburn_coeff_TL=[.023, .8, .33]  tube_roughness_heat_TL=15e-6 m  tube_Re_lam_heat_TL=2000  tube_Re_tur_heat_TL=4000  tube_Nu_lam_generic_TL=3.66  bank_arrangement_TL=fluids.heat_exchangers.enum.BankArrangement.Inline  bank_num_rows_TL=5  bank_tubes_per_row_TL=5  bank_width_TL=1 m  bank_tube_diameter_TL=0.05 m  bank_longitudinal_pitch_TL=0.15 m  bank_transverse_pitch_TL=0.15 m  bank_pressure_loss_spec_TL=fluids.heat_exchangers.enum.BankPressureLossSpec.Martin  bank_euler_TL=10  bank_heat_coeff_spec_TL=fluids.heat_exchangers.enum.BankHeatCoeffSpec.Martin  bank_colburn_coeff_TL=[.27, .63, .36]  generic_flow_area_TL=0.01 m^2  generic_heat_area_TL=2 m^2  generic_volume_TL=0.05 m^3  generic_loss_coeff_TL=10  generic_colburn_coeff_TL=[.023, .8, .33]  fouling_factor_TL=PlntThrRadCoolFoul m^2*K/kW  fin_area_TL=0 m^2  fin_efficiency_TL=0  p_init_TL=EnvAbsPrs Pa  T_init_TL=EnvAirTemp K  flow_geometry_MA=fluids.heat_exchangers.enum.FlowGeometryMA.Generic  tube_num_MA=1  tube_length_MA=5 m  tube_cross_section_MA=fluids.heat_exchangers.enum.TubeCrossSection.Circular  tube_diameter_MA=0.1 m  tube_width_MA=0.1 m  tube_height_MA=0.1 m  tube_inner_diameter_MA=0.05 m  tube_outer_diameter_MA=0.1 m  tube_flow_area_MA=0.01 m^2  tube_wetted_perimeter_MA=0.4 m  tube_heat_perimeter_MA=0.4 m  tube_pressure_loss_spec_MA=fluids.heat_exchangers.enum.TubePressureLossSpec.Haaland  tube_loss_coeff_MA=10  tube_local_pressure_loss_spec_MA=fluids.heat_exchangers.enum.LocalLossSpec.AggregateLength  tube_length_add_MA=0.1 m  tube_local_loss_coefficient_MA=0.1  tube_roughness_pressure_MA=15e-6 m  tube_Re_lam_pressure_MA=2000  tube_Re_tur_pressure_MA=4000  tube_shape_factor_generic_MA=64  tube_heat_coeff_spec_MA=fluids.heat_exchangers.enum.TubeHeatCoeffSpec.Gneilinski  tube_colburn_coeff_MA=[.023, .8, .33]  tube_roughness_heat_MA=15e-6 m  tube_Re_lam_heat_MA=2000  tube_Re_tur_heat_MA=4000  tube_Nu_lam_generic_MA=3.66  bank_arrangement_MA=fluids.heat_exchangers.enum.BankArrangement.Inline  bank_num_rows_MA=5  bank_tubes_per_row_MA=5  bank_width_MA=1 m  bank_tube_diameter_MA=0.05 m  bank_longitudinal_pitch_MA=0.15 m  bank_transverse_pitch_MA=0.15 m  bank_pressure_loss_spec_MA=fluids.heat_exchangers.enum.BankPressureLossSpec.Martin  bank_euler_MA=10  bank_heat_coeff_spec_MA=fluids.heat_exchangers.enum.BankHeatCoeffSpec.Martin  bank_colburn_coeff_MA=[.27, .63, .36]  generic_flow_area_MA=PlntThrRadAirAreaFlw m^2  generic_heat_area_MA=PlntThrRadAirAreaPr m^2  generic_volume_MA=PlntThrRadMoistAirVol m^3  generic_loss_coeff_MA=10  generic_colburn_coeff_MA=[0.27, 0.63, 0.36]  fouling_factor_MA=PlntThrRadAirFoul m^2*K/kW  fin_area_MA=PlntThrRadAirAreaFins m^2  fin_efficiency_MA=PlntThrRadFinEff  p_init_MA=EnvAbsPrs Pa  T_init_MA=EnvAirTemp K  humidity_spec_MA=foundation.enum.HumiditySpec.RelativeHumidity  RH_init_MA=PlntThrCabRelHInit  x_w_init_MA=0.01  y_w_init_MA=0.01  HR_init_MA=0.01  Tw_init_MA=287 K  trace_gas_spec_MA=foundation.enum.trace_gas_spec.mole_fraction  x_g_init_MA=0.001  y_g_init_MA=PlntThrCabCO2Init  r_d_init_MA=0  RH_ws_MA=1  time_constant_cond_MA=1e-3 s  time_constant_evap_MA=1e-3 s  fraction_entrained_MA=1
  Simulink-PS Converter : nesl_utility/Simulink-PS Converter  PhysicalDomain=network_engine_domain  SubClassName=ps_input  LeftPortType=input  RightPortType=output  PseudoPeriodic=off  Frequencies=[]  NoiseDistribution=none  NoiseParameters=[]  Unit=rpm  AffineConversion=off  FilteringAndDerivatives=provide  SimscapeFilterOrder=1  InputFilterTimeConstant=0.001  UdotUserProvided=0
  Simulink-PS Converter5 : nesl_utility/Simulink-PS Converter  PhysicalDomain=network_engine_domain  SubClassName=ps_input  LeftPortType=input  RightPortType=output  PseudoPeriodic=off  Frequencies=[]  NoiseDistribution=none  NoiseParameters=[]  Unit=K  AffineConversion=on  FilteringAndDerivatives=provide  SimscapeFilterOrder=1  InputFilterTimeConstant=0.001  UdotUserProvided=0
  Simulink-PS Converter6 : nesl_utility/Simulink-PS Converter  PhysicalDomain=network_engine_domain  SubClassName=ps_input  LeftPortType=input  RightPortType=output  PseudoPeriodic=off  Frequencies=[]  NoiseDistribution=none  NoiseParameters=[]  Unit=Pa  AffineConversion=off  FilteringAndDerivatives=provide  SimscapeFilterOrder=1  InputFilterTimeConstant=0.001  UdotUserProvided=0
  Simulink-PS Converter7 : nesl_utility/Simulink-PS Converter  PhysicalDomain=network_engine_domain  SubClassName=ps_input  LeftPortType=input  RightPortType=output  PseudoPeriodic=off  Frequencies=[]  NoiseDistribution=none  NoiseParameters=[]  Unit=1  AffineConversion=off  FilteringAndDerivatives=provide  SimscapeFilterOrder=1  InputFilterTimeConstant=0.001  UdotUserProvided=0
  Simulink-PS Converter8 : nesl_utility/Simulink-PS Converter  PhysicalDomain=network_engine_domain  SubClassName=ps_input  LeftPortType=input  RightPortType=output  PseudoPeriodic=off  Frequencies=[]  NoiseDistribution=none  NoiseParameters=[]  Unit=1  AffineConversion=off  FilteringAndDerivatives=provide  SimscapeFilterOrder=1  InputFilterTimeConstant=0.001  UdotUserProvided=0
  B : PMIOPort  Side=Left
  C : PMIOPort  Port=2  Side=Left
  A : PMIOPort  Port=3  Side=Right
  01 : Outport
  wires:
  Product/1 -> 01/1  "FanPwr"
  Gain/1 -> Product/1
  PS-Simulink Converter/1 -> Product/2
  2/1 -> LPF with IC1/1(u)
  LPF with IC1/1(y) -> Max Speed [rpm]/1
  1/1 -> Bus Selector1/1
  Bus Selector1/4 -> Simulink-PS Converter8/1  "<CO2Init>"
  Bus Selector1/1 -> Simulink-PS Converter5/1  "<AmbTemp>"
  Bus Selector1/2 -> Simulink-PS Converter6/1  "<BaroPress>"
  Bus Selector1/3 -> Simulink-PS Converter7/1  "<RelHumidity>"
  Max Speed [rpm]/1 -> Simulink-PS Converter/1, Gain/1
  connections:
  PS-Simulink Converter/LConn1 -- Ideal Torque Sensor/RConn2
  Ideal Torque Sensor/RConn1 -- Fan/RConn2
  Ideal Torque Sensor/LConn1 -- Ideal Angular Velocity Source/LConn1
  Environment Air1/LConn1 -- Fan/RConn1
  Environment Air1/RConn2 -- Simulink-PS Converter6/RConn1
  Environment Air1/RConn1 -- Simulink-PS Converter5/RConn1
  Environment Air1/RConn4 -- Simulink-PS Converter8/RConn1
  Environment Air1/RConn3 -- Simulink-PS Converter7/RConn1
  B/RConn1 -- Radiator/LConn2
  Radiator/LConn1 -- Coolant Properties/RConn1 -- A/RConn1
  Radiator/RConn2 -- C/RConn1
  Fan/LConn1 -- Radiator/RConn1
  Fan/LConn2 -- Ideal Angular Velocity Source/RConn2 -- Mechanical Rotational Reference/LConn1
  Simulink-PS Converter/RConn1 -- Ideal Angular Velocity Source/RConn1
